simulink model "SimLink01"  (R2021a)
settings: Solver=FixedStepDiscrete  StartTime=0.0  StopTime=4  RelTol=1e-3
libraries: dsparch4 x2, dspsrcs4 x1
settings Model: Creator=lefs3303  LastModifiedBy=lefs3303

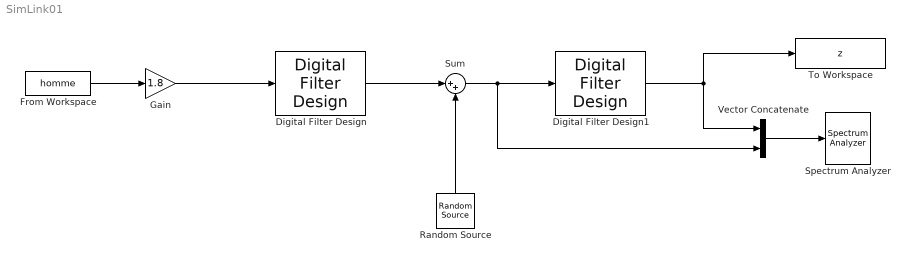
== system SimLink01 ==
  Digital Filter Design : dsparch4/Digital Filter Design  mwdsp_browser_bugfix_var=off
  Digital Filter Design1 : dsparch4/Digital Filter Design  mwdsp_browser_bugfix_var=off
  From Workspace : FromWorkspace  VariableName=homme  SampleTime=1/16000
  Gain : Gain  Gain=1.8
  Random Source : dspsrcs4/Random Source  SrcType=Gaussian  NormMethod=Ziggurat  CltLength=12  MinVal=0  MaxVal=1  MeanVal=0  VarVal=0.048  RepMode=Not repeatable  rawSeed=1  IsInherit=off  SampMode=Discrete  SampTime=1/16000  SampFrame=1  DataType=Double  OutComplex=Real  OutputFrames=off
  Spectrum Analyzer : SpectrumAnalyzer
  Sum : Sum  Inputs=|++
  To Workspace : ToWorkspace  VariableName=z  SampleTime=-1
      settings: Save2DSignal=2-D array (concatenate along first dimension)
  Vector Concatenate : Concatenate  Mode=Multidimensional array  ConcatenateDimension=2
  wires:
  From Workspace/1 -> Gain/1
  Gain/1 -> Digital Filter Design/1
  Vector Concatenate/1 -> Spectrum Analyzer/1
  Digital Filter Design1/1 -> Vector Concatenate/1, To Workspace/1
  Digital Filter Design/1 -> Sum/1
  Random Source/1 -> Sum/2
  Sum/1 -> Vector Concatenate/2, Digital Filter Design1/1
